simulink model "quadcopter_temp"  (R2023b)
settings: Solver=ode3  StartTime=0  StopTime=60  FixedStep=0.005  RelTol=1e-3  EnableMultiTasking=on
values from neighbouring files (symbols this model uses):
  alpha_x = Bmatrix\BCx    [variables.m]
  alpha_y = Bmatrix\BCy    [variables.m]
  alpha_z = Bmatrix\BCz    [variables.m]
  g = 9.81    [variables.m]
  I_c = [ ... (first row only)    [variables.m]
  M_rb = [total_mass*eye(3),zeros(3,3) ... (first row only)    [variables.m]
  total_mass = 1    [variables.m]
undefined symbols (not defined in the file or in its folder): motor_thrust, tilt_force_length
libraries: simulink_extras x7, slpidlib x6, dspsigops x3, simulink x3, aerolibutil x2, vrlib x1
(part 2 of 2)

== system quadcopter_temp/Sudo-Random-Movement/Smoothing (fast->slow)2/For Each Subsystem ==
  u : Inport  Partition=on  PartitionDimension=1  PartitionWidth=1  PartitionOffset=0
  For Each : ForEach  DisableCoverage=on
  Gain : Gain  Gain=1/nSmooth
  Sum of Elements : Sum  Inputs=+
  Tapped Delay : simulink/Discrete/Tapped Delay  vinit=mean(smoothing0)  samptime=h1  NumDelays=nSmooth  DelayOrder=Oldest  includeCurrent=off
  y : Outport  ConcatenationDimension=1
  wires:
  u/1 -> Tapped Delay/1
  Sum of Elements/1 -> Gain/1
  Tapped Delay/1 -> Sum of Elements/1
  Gain/1 -> y/1

== matlab function quadcopter_temp/Outer loop position control/MATLAB Function ==
  data: Deltap_e input; Deltap_b output; psi input
function Deltap_b = fcn(Deltap_e,psi)

R = [ cos(psi) , -sin(psi) ;
      sin(psi) ,  cos(psi) ];

Deltap_b = R'*Deltap_e;

== matlab function quadcopter_temp/Quadcopter model/Drone/MATLAB Function ==
  data: nu input; Cnunu output; m input; Ic input
function Cnunu = fcn(nu,m,Ic)

v = nu(1:3);  % linear velocities (expressed in the body frame)
omega = nu(4:6); % angular velocities (expressed in the body frame)


Cnunu = [ cross(omega,m*v) ; -cross(Ic*omega,omega) ];

== matlab function quadcopter_temp/Desired trajectory/pd(sigma) ==
  data: alpha_x input; pd output; alpha_y input; alpha_z input; sigma input
function pd = fcn(alpha_x,alpha_y,alpha_z,sigma)

if sigma<1
    alphax = alpha_x(1:4);
    alphay = alpha_y(1:4);
    alphaz = alpha_z(1:4);
elseif sigma<2
    alphax = alpha_x(5:8);
    alphay = alpha_y(5:8);
    alphaz = alpha_z(5:8);
else
    alphax = alpha_x(9:12);
    alphay = alpha_y(9:12);
    alphaz = alpha_z(9:12);
end

% Added a negative on the Z to make sure it is not going underground
if sigma<3
    pd = [ b(sigma)'*alphax ; b(sigma)'*alphay ; -b(sigma)'*alphaz];
else % stay on the last waypoint at the end of the path
    pd = [ b(3)'*alphax ; b(3)'*alphay ; -b(3)'*alphaz]; 
end

end

%-------------------------
function b_out = b(sigma)

b_out = [ 1 ; sigma ; sigma^2 ; sigma^3 ];

end

== matlab function quadcopter_temp/Quadcopter model/Drone/MATLAB Function1 ==
  data: R_be output; nu input; eta input; eta_dot output
function [R_be,eta_dot]= J_Theta(nu, eta)

% Euler angle extraction
phi = eta(4);
theta = eta(5);
psi = eta(6);

R_xphi = [ 1 0 0 ; 0 cos(phi) -sin(phi) ; 0 sin(phi) cos(phi) ];
R_ytheta = [ cos(theta) 0 sin(theta) ; 0 1 0 ; -sin(theta) 0 cos(theta) ];
R_zpsi = [ cos(psi) -sin(psi) 0 ; sin(psi) cos(psi) 0 ; 0 0 1 ];

% rotation matrix
R_be = R_zpsi * R_ytheta * R_xphi;

% angular velocity transformation
T_Theta = [ 1 sin(phi)*tan(theta) cos(phi)*tan(theta) ; 0 cos(phi) -sin(phi) ; 0 sin(phi)/cos(theta) cos(phi)/cos(theta) ];

J_Theta = [ R_be , zeros(3) ; zeros(3) , T_Theta ];

eta_dot = J_Theta*nu;

== matlab function quadcopter_temp/Desired trajectory/sigma_dot ==
  data: alpha_x input; sigma_dot output; alpha_y input; alpha_z input; rhod input; sigma input
function sigma_dot = fcn(alpha_x,alpha_y,alpha_z,rhod,sigma)


if sigma<1
    alphax = alpha_x(1:4);
    alphay = alpha_y(1:4);
    alphaz = alpha_z(1:4);
elseif sigma<2
    alphax = alpha_x(5:8);
    alphay = alpha_y(5:8);
    alphaz = alpha_z(5:8);
else
    alphax = alpha_x(9:12);
    alphay = alpha_y(9:12);
    alphaz = alpha_z(9:12);
end

xdp = b_prime(sigma)'*alphax;
ydp = b_prime(sigma)'*alphay;
zdp = b_prime(sigma)'*alphaz;

sigma_dot = rhod / sqrt(xdp^2+ydp^2+zdp^2);

end



%-------------------------
function bp_out = b_prime(sigma)

bp_out = [ 0 ; 1 ; 2*sigma ; 3*sigma^2 ];

end

== matlab function quadcopter_temp/MATLAB Function ==
  data: contact input; ref_in input; eta input; ref_out output; mem_in input; mem_out output
function [ref_out,mem_out]= fcn(contact,ref_in,eta,mem_in)


if contact == 0
    ref_out = ref_in;
    mem_out = -1;
else

    %OMG Contact!
    
    %Test if altitude is high enough for drop. Else move sideways! 
    if -1* eta(3) < 50
        mem_out = 0;
    else
        mem_out = 1;
    end
    if mem_in == 0
        ref_out = [-500;0;0;0];
    elseif mem_in == 1
        ref_out = [-50;0;0;0];
        if eta(3) < -60
            ref_out = [-50;0;0;0];
        end
    else
        ref_out = ref_in;
    end
end
